simulink model "control"  (R2021b)
settings: Solver=VariableStepAuto  StartTime=0.0  StopTime=4  RelTol=1e-3
values from neighbouring files (symbols this model uses):
  q0 = [-0.9273 -1.287 0.7 2.2143]    [generated_traj.mat]    (also in init_traj.m = [-0.9273;-1.2870;0.7000;2.2143])
  Tc = 0.001    [generated_traj.mat]    (also in init_traj.m)
undefined symbols (not defined in the file or in its folder): DiscIntNeverNeededParam
settings Model: Creator=patlee  LastModifiedBy=patlee

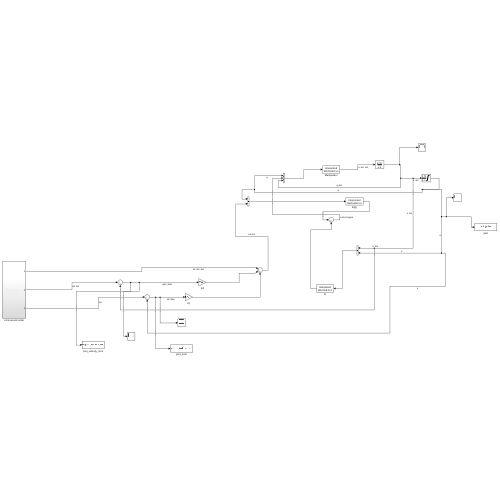
[thumbnail: Simulink's stored preview of the top-level diagram]
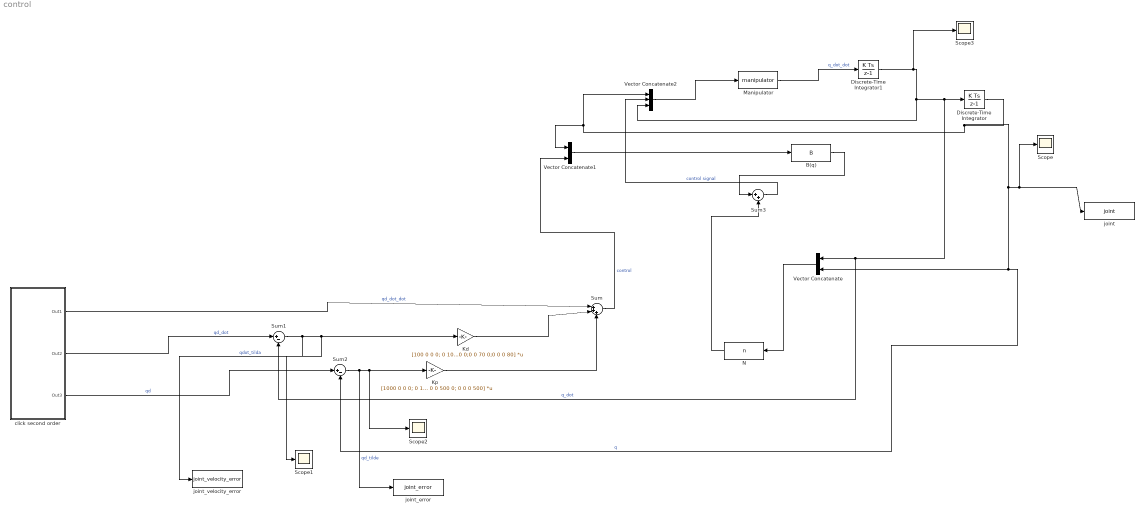
== system control ==
  B(q) : MATLABFcn  MATLABFcn=B  OutputDimensions=4
  Discrete-Time Integrator : DiscreteIntegrator  InitialCondition=q0  SampleTime=Tc  LimitOutput=on  UpperSaturationLimit=[inf;inf;inf;inf]  LowerSaturationLimit=[-inf;-inf;-inf;-inf]  ICPrevOutput=DiscIntNeverNeededParam  ICPrevScaledInput=DiscIntNeverNeededParam
  Discrete-Time Integrator1 : DiscreteIntegrator  InitialCondition=[0;0;0;0]  SampleTime=0.001  ICPrevOutput=DiscIntNeverNeededParam  ICPrevScaledInput=DiscIntNeverNeededParam
  Kd : Gain  Gain=[100 0 0 0; 0 100 0 0;0 0 70 0;0 0 0 80]  Multiplication=Matrix(K*u)
  Kp : Gain  Gain=[1000 0 0 0; 0 1000 0 0; 0 0 500 0; 0 0 0 500]  Multiplication=Matrix(K*u)
  Manipulator : MATLABFcn  MATLABFcn=manipulator  OutputDimensions=4
  N : MATLABFcn  MATLABFcn=n  OutputDimensions=4
  Scope{,1..3} (4 alike) : Scope
  Sum : Sum  Inputs=|+++
  Sum1 : Sum  Inputs=|+-
  Sum2 : Sum  Inputs=|+-
  Sum3 : Sum  Inputs=|++
  Vector Concatenate : Concatenate
  Vector Concatenate1 : Concatenate
  Vector Concatenate2 : Concatenate  NumInputs=3
  click second order : Subsystem
  joint : ToWorkspace  VariableName=joint  SampleTime=0.001
  joint_error : ToWorkspace  VariableName=joint_error  SampleTime=-1
  joint_velocity_error : ToWorkspace  VariableName=joint_velocity_error  SampleTime=-1
  wires:
  click second order/1(Out1) -> Sum/1  "qd_dot_dot"
  click second order/2(Out2) -> Sum1/1  "qd_dot"
  click second order/3(Out3) -> Sum2/1  "qd"
  Discrete-Time Integrator1/1 -> Scope3/1, Vector Concatenate2/3, Sum1/2, Vector Concatenate/1, Discrete-Time Integrator/1  "q_dot"
  Sum1/1 -> Scope1/1, joint_velocity_error/1, Kd/1  "qdot_tilda"
  Sum2/1 -> joint_error/1, Scope2/1, Kp/1  "qd_tilde"
  Kd/1 -> Sum/2
  Kp/1 -> Sum/3
  Sum/1 -> Vector Concatenate1/2  "control"
  B(q)/1 -> Sum3/1
  N/1 -> Sum3/2
  Sum3/1 -> Vector Concatenate2/2  "control signal"
  Manipulator/1 -> Discrete-Time Integrator1/1  "q_dot_dot"
  Discrete-Time Integrator/1 -> Sum2/2, Vector Concatenate/2, Scope/1, joint/1, Vector Concatenate2/1, Vector Concatenate1/1  "q"
  Vector Concatenate/1 -> N/1
  Vector Concatenate1/1 -> B(q)/1
  Vector Concatenate2/1 -> Manipulator/1

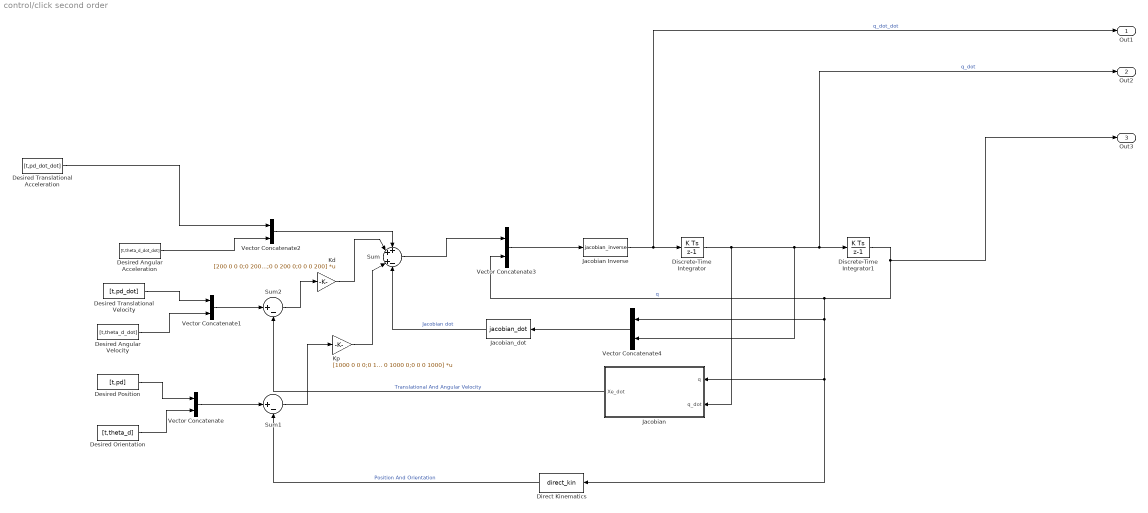
== system control/click second order ==
  Desired Angular Acceleration : FromWorkspace  VariableName=[t,theta_d_dot_dot]
  Desired Angular Velocity : FromWorkspace  VariableName=[t,theta_d_dot]
  Desired Orientation : FromWorkspace  VariableName=[t,theta_d]
  Desired Position : FromWorkspace  VariableName=[t,pd]
  "Desired Translational Acceleration " : FromWorkspace  VariableName=[t,pd_dot_dot]
  Desired Translational Velocity : FromWorkspace  VariableName=[t,pd_dot]
  Direct Kinematics : MATLABFcn  MATLABFcn=direct_kin  OutputDimensions=4
  Discrete-Time Integrator : DiscreteIntegrator  InitialCondition=[0;0;0;0]  SampleTime=Tc  ICPrevOutput=DiscIntNeverNeededParam  ICPrevScaledInput=DiscIntNeverNeededParam
  Discrete-Time Integrator1 : DiscreteIntegrator  InitialCondition=q0  SampleTime=Tc  ICPrevOutput=DiscIntNeverNeededParam  ICPrevScaledInput=DiscIntNeverNeededParam
  "Jacobian " : MATLAB Function  TreatAsAtomicUnit=on
  Jacobian Inverse : MATLABFcn  MATLABFcn=jacobian_inverse  OutputDimensions=4
  Jacobian_dot : MATLABFcn  MATLABFcn=jacobian_dot  OutputDimensions=4
  Kd : Gain  Gain=[200 0 0 0;0 200 0 0;0 0 200 0;0 0 0 200]  Multiplication=Matrix(K*u)
  Kp : Gain  Gain=[1000 0 0 0;0 1000 0 0;0 0 1000 0;0 0 0 1000]  Multiplication=Matrix(K*u)
  Sum : Sum  Inputs=++|+-
  Sum1 : Sum  Inputs=|+-
  Sum2 : Sum  Inputs=|+-
  Vector Concatenate{,1..4} (5 alike) : Concatenate
  Out1 : Outport
  Out2 : Outport  Port=2
  Out3 : Outport  Port=3
  wires:
  Sum1/1 -> Kp/1
  Desired Angular Acceleration/1 -> Vector Concatenate2/2
  Sum2/1 -> Kd/1
  Desired Angular Velocity/1 -> Vector Concatenate1/2
  Jacobian_dot/1 -> Sum/4  "Jacobian dot"
  Vector Concatenate1/1 -> Sum2/1
  Vector Concatenate/1 -> Sum1/1
  Desired Orientation/1 -> Vector Concatenate/2
  Discrete-Time Integrator1/1 -> Vector Concatenate3/2, Vector Concatenate4/1, Direct Kinematics/1, "Jacobian "/1(q), Out3/1  "q"
  Sum/1 -> Vector Concatenate3/1
  Jacobian Inverse/1 -> Out1/1, Discrete-Time Integrator/1  "q_dot_dot"
  Vector Concatenate3/1 -> Jacobian Inverse/1
  Kp/1 -> Sum/3
  Vector Concatenate4/1 -> Jacobian_dot/1
  "Desired Translational Acceleration "/1 -> Vector Concatenate2/1
  Discrete-Time Integrator/1 -> "Jacobian "/2(q_dot), Vector Concatenate4/2, Out2/1, Discrete-Time Integrator1/1  "q_dot"
  Vector Concatenate2/1 -> Sum/1
  Desired Translational Velocity/1 -> Vector Concatenate1/1
  Kd/1 -> Sum/2
  Desired Position/1 -> Vector Concatenate/1
  Direct Kinematics/1 -> Sum1/2  "Position And Orientation"
  "Jacobian "/1(Xe_dot) -> Sum2/2  "Translational And Angular Velocity"

== matlab function control/click second order/Jacobian  ==
  data: q input; Xe_dot output; q_dot input
function Xe_dot= fcn(q,q_dot)


    theta1=q(1);
    theta2=q(2);
    
    a1=0.5;
    
    a2=0.5;
    
    Jacobian=[- a2*sin(theta1 + theta2) - a1*sin(theta1), -a2*sin(theta1 + theta2), 0, 0; 
        a2*cos(theta1 + theta2) + a1*cos(theta1), a2*cos(theta1 + theta2), 0,0; 
        0, 0, -1, 0;
        1, 1, 0, 1];
    
    Xe_dot=Jacobian*q_dot;

end
